simulink model "design_lqr"  (R2019b)
settings: Solver=VariableStepAuto  StartTime=0.0  StopTime=10  RelTol=1e-3
values from neighbouring files (symbols this model uses):
  Ac = [A-B*F B*F;zeros(1*9) A-Ke*C1]    [design_hinfinity.m]    (also in design_lqr_m.m = [A-B*F B*F;zeros(9) A-Ke*C1]; design_v1.m)
  Bc = 1.0e+03*[ ... (first row only)    [design_hinfinity.m]    (also in design_lqr_m.m = [B*G;Zero_tem]; design_v1.m)
  Cc = [ 1     0     0     0     0     0     0     0     0  0     0     0     0     0     0     0     0     0 ... (first row only)    [design_hinfinity.m]    (also in design_lqr_m.m = [C1 zeros(9)]; design_v1.m)
  Vw = [ ... (first row only)    [design_hinfinity.m]    (also in design_lqr_m.m = [E;E]; design_v1.m = [E;E-Ke*[0;0;1;1;0;0;1;0;0]])
  x0 = [0 0 0 0 0 0 0 0 0;0 -0.1 0 0 0 0 0 0 0;0 0 0 0 0 0 0 0 0;0 0 0 0 0 0 0 0 0;0 0 0 0 0 0 0 0 0;0 0 0 0 0 0 0 0 0;0 0 0 0 0 0 0 0 0;0 0 0 0 0 0 0 0 0;0 0 0 0 0 0 0 0  0.1;0 0 0 0 0 0 0 0 0  ;      0 0 0 0 0 0 0 0 0  ;      0 0 0 0 0 0 0 0 0 ;0 0 0 0 0 0 0 0 0   ;      0 0 0 0 0 0 0 0 0    ;     0 0 0 0 0 0 0 0 0;0 0 0 0 0 0 0 0 0;0 0 0 0 0 0 0 0 0;0 0 0 0 0 0 0 0 0]    [design_hinfinity.m]    (also in design_lqr_m.m = [0;-0.1;0;0;0;0;0;0;0.1;0;0;0;0;0;0;0;0;0]; design_v1.m = [0;-0.1;0;0;0;0;0;0;0.1;0;0;0;0;0;0;0;0;0])
libraries: simulink x2
settings Model: Creator=50474  LastModifiedBy=Administrator
settings DataIOCC: ReturnWorkspaceOutputs=off
settings DebuggingCC: ArithmeticOperatorsInVariantConditions=warning
settings SFSimCC: SimUseLocalCustomCode=off  CustomCodeUndefinedFunction=UseInterfaceOnly
settings RTWCC: RTWUseLocalCustomCode=off

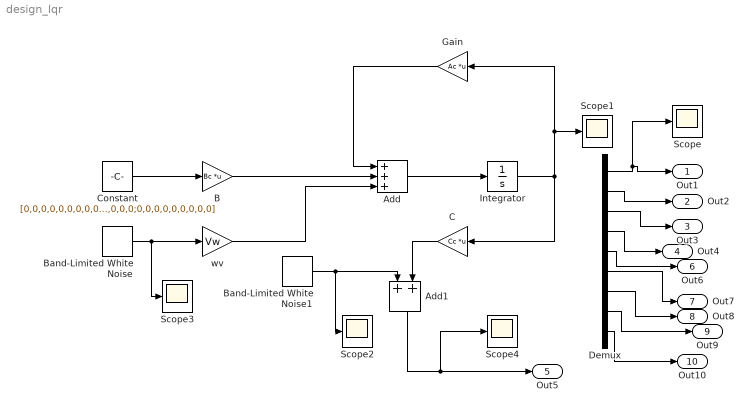
== system design_lqr ==
  Add : Sum  Inputs=+++
  Add1 : Sum
  B : Gain  Gain=Bc  Multiplication=Matrix(K*u)
  Band-Limited White Noise : simulink/Sources/Band-Limited White Noise  Cov=0.00001  Ts=0.001  seed=[23341]
  Band-Limited White Noise1 : simulink/Sources/Band-Limited White Noise  Cov=[0.00001]  Ts=0.001  seed=[23341]
  C : Gain  Gain=Cc  Multiplication=Matrix(K*u)
  Constant : Constant  Value=[0,0,0,0,0,0,0,0,0;0,0,0,0,0,0,0,0,0;0,0,0,0,0,0,0,0,0]
  Demux : Demux  Outputs=9
  Gain : Gain  Gain=Ac  Multiplication=Matrix(K*u)
  Integrator : Integrator  InitialCondition=x0
  Scope{,1..4} (5 alike) : Scope
  wv : Gain  Gain=Vw
  Out1 : Outport  VectorParamsAs1DForOutWhenUnconnected=off
  Out2 : Outport  Port=2  VectorParamsAs1DForOutWhenUnconnected=off
  Out3 : Outport  Port=3  VectorParamsAs1DForOutWhenUnconnected=off
  Out4 : Outport  Port=4  VectorParamsAs1DForOutWhenUnconnected=off
  Out5 : Outport  Port=5  SignalName=y  VectorParamsAs1DForOutWhenUnconnected=off
  Out6 : Outport  Port=6  VectorParamsAs1DForOutWhenUnconnected=off
  Out7 : Outport  Port=7  VectorParamsAs1DForOutWhenUnconnected=off
  Out8 : Outport  Port=8  VectorParamsAs1DForOutWhenUnconnected=off
  Out9 : Outport  Port=9  VectorParamsAs1DForOutWhenUnconnected=off
  Out10 : Outport  Port=10  VectorParamsAs1DForOutWhenUnconnected=off
  wires:
  Add/1 -> Integrator/1
  Integrator/1 -> Scope1/1, Gain/1, C/1
  Gain/1 -> Add/1
  Constant/1 -> B/1
  B/1 -> Add/2
  wv/1 -> Add/3
  Band-Limited White Noise/1 -> Scope3/1, wv/1
  C/1 -> Add1/2
  Band-Limited White Noise1/1 -> Scope2/1, Add1/1
  Demux/1 -> Scope/1, Out1/1
  Demux/2 -> Out2/1
  Demux/3 -> Out3/1
  Demux/4 -> Out4/1
  Add1/1 -> Scope4/1, Out5/1
  Demux/5 -> Out6/1
  Demux/6 -> Out7/1
  Demux/7 -> Out8/1
  Demux/8 -> Out9/1
  Demux/9 -> Out10/1
